simulink model "FirstCode_Control"  (R2014b)
settings: configuration reference "Embedded_Configuration" (kept outside this file)
PostLoadFcn:
  | c2000demoscallback(1)
settings Model: Creator=The MathWorks Inc.  LastModifiedBy=Nathan

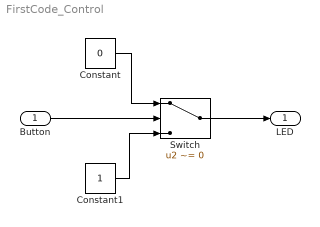
== system FirstCode_Control ==
  Button : Inport  OutDataTypeStr=int16
  Constant : Constant  Value=0
  Constant1 : Constant
  Switch : Switch  Criteria=u2 ~= 0  OutDataTypeStr=int16
  LED : Outport  OutDataTypeStr=int16
  wires:
  Button/1 -> Switch/2
  Switch/1 -> LED/1
  Constant/1 -> Switch/1
  Constant1/1 -> Switch/3
